simulink model "threephase3level_SVPWM_Bidirectional_C"  (R2024a)
settings: Solver=ode4  StartTime=0.0  StopTime=0.5  FixedStep=1e-6  MaxStep=0.00001  MinStep=0.000001  RelTol=1e-3  EnableMultiTasking=on
libraries: spsIGBTDiodeLib x12, spsDiodeLib x6, spsVoltageMeasurementLib x6, slpidlib x4, spsACVoltageSourceLib x3, spsSeriesRLCBranchLib x3, spsabctoAlphaBetaZeroLib x2, spsAlphaBetaZerotodq0Lib x1, spsControlledVoltageSourceLib x1, spsCurrentMeasurementLib x1, spsGroundLib x1, simulink x1
settings Model: Creator=hp  LastModifiedBy=rkavi
settings SolverCC: ZeroCrossControl=DisableAll  AlgebraicLoopSolver=TrustRegion
settings DataIOCC: LimitDataPoints=on  SaveFormat=Array  ReturnWorkspaceOutputs=off
settings OptimizationCC: LifeSpan=inf
settings DebuggingCC: UnconnectedInputMsg=warning  UnconnectedOutputMsg=warning  UnconnectedLineMsg=warning  SFUnexpectedBacktrackingDiag=warning  SFNoUnconditionalDefaultTransitionDiag=warning  ArithmeticOperatorsInVariantConditions=warning
settings HardwareCC: ProdBitPerPointer=32  ProdBitPerSizeT=32  ProdBitPerPtrDiffT=32  ProdLargestAtomicFloat=None  ProdIntDivRoundTo=Undefined  ProdEndianess=Unspecified  ProdWordSize=32  ProdHWDeviceType=32-bit Generic
settings ModelReferenceCC: EnableRefExpFcnMdlSchedulingChecks=on  PropagateSignalLabelsOutOfModel=off
settings SFSimCC: SimUseLocalCustomCode=off  CustomCodeUndefinedFunction=UseInterfaceOnly
settings RTWCC: RTWUseLocalCustomCode=off  GPUComputeCapability=3.5
settings CodeAppCC: StateflowObjectComments=on
settings GRTTargetCC: TargetLangStandard=C89/C90 (ANSI)
settings ConfigComp: CovMetricSettings=dw  CovSaveCumulativeToWorkspaceVar=on  CovSaveSingleToWorkspaceVar=on  CovExternalEMLEnable=off
settings SimscapeCC: SimscapeNormalizeSystem=off

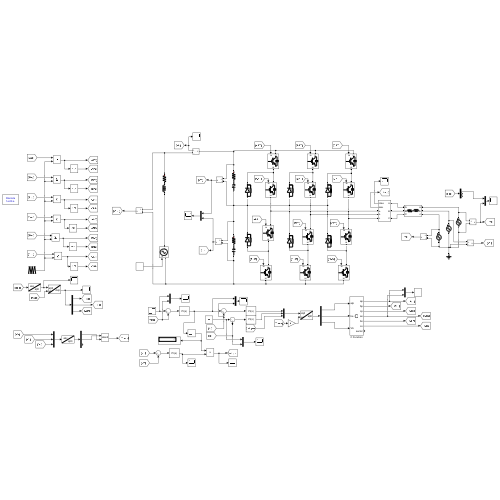
[thumbnail: Simulink's stored preview of the top-level diagram]
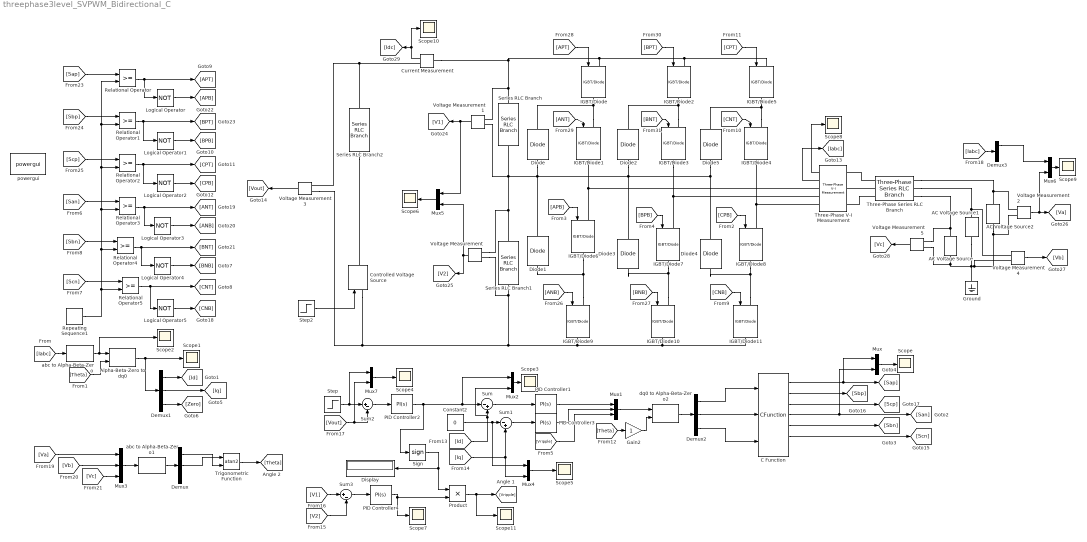
== system threephase3level_SVPWM_Bidirectional_C ==
  AC Voltage Source : spsACVoltageSourceLib/AC Voltage Source  Amplitude=325  Phase=240  Frequency=50  SampleTime=0  Measurements=None  BusType=swing  Pref=10e3  Qref=0  Qmin=-inf  Qmax=+inf
  AC Voltage Source1 : spsACVoltageSourceLib/AC Voltage Source  Amplitude=325  Phase=120  Frequency=50  SampleTime=0  Measurements=None  BusType=swing  Pref=10e3  Qref=0  Qmin=-inf  Qmax=+inf
  AC Voltage Source2 : spsACVoltageSourceLib/AC Voltage Source  Amplitude=325  Phase=0  Frequency=50  SampleTime=0  Measurements=None  BusType=swing  Pref=10e3  Qref=0  Qmin=-inf  Qmax=+inf
  Alpha-Beta-Zero to dq0 : spsAlphaBetaZerotodq0Lib/Alpha-Beta-Zero to dq0  Alignment=Aligned with phase A axis
  C Function : CFunction  OutputCode=|  CodegenOutputCode=|
      OutputCode=|
      | float sec_a=0,sec_b=0,sec_c=0;
      | 	float t_o = 0,ta = 0,tb = 0,tc = 0,tsec = 0;
      | 
      |     sec_a = be;										//Beta;
      | 	sec_b = ((-be/2)+(alp*0.866));			//(-0.5*Beta+(0.866*alpha));
      | 	sec_c = ((-be/2)-(alp*0.866));			//(-0.5*Beta-(0.866*alpha));
      |     
      |     if(sec_a>=0)
      |      {
      |          if(sec_b>=0)
      |        	  {											//	sector 1
      |     		t_o = ((1 - (sec_a+sec_b))/2)-Vb;							//	t_1 = sec_b, t_2 =sec_a
      |     		ta = sec_a+sec_b+(t_o);
      |     		tb  = sec_a+(t_o);
      |     		tc  = (t_o);
      |             tsec = 1;
      |          }
      |        else
      |          {
      |             if(sec_c>=0)												//	sector 3
      |         	{
      |             	t_o = ((1 - (sec_a+sec_c))/2)-Vb;						//	t_1 = sec_a, t_2 =sec_c
      |         		ta = (t_o);
      |         		tb = sec_a+sec_c+(t_o);
      |         		tc = sec_c+(t_o);
      |                 tsec = 3;
      |              }
      |             else
      |             {                                                        //	sector 2
      |         		t_o = ((1 + (sec_c+sec_b))/2)-Vb;					//	t_1 = -sec_c, t_2 =-sec_b
      |         		ta = -sec_c+(t_o);
      |         		tb = -(sec_c+sec_b)+(t_o);
      |         		tc = (t_o);
      |                 tsec = 2;
      |             }
      |        }
      |      }
      |     else
      |        {
      |          if(sec_b>=0)
      |            {
      |                if(sec_c>=0)                                                  //	sector 5
      |         		{
      |                     t_o = ((1 - (sec_c+sec_b))/2)-Vb; 				//	t_1 = sec_c, t_2 =sec_b
      |         		    ta = sec_b+(t_o);
      |         		    tb = (t_o);
      |         		    tc = sec_c+sec_b+(t_o);
      |                     tsec = 5;    
      |                 }
      |            else                                                  //	sector 6
      |         		{
      |                     t_o = ((1 + (sec_a+sec_c))/2)-Vb; 				//	t_1 = -sec_a, t_2 =-sec_c
      |         		    ta = -(sec_a+sec_c)+(t_o);
      |         		    tb = (t_o);
      |         		    tc = -sec_a+(t_o);
      |                     tsec = 6;
      |                 }
      |         }
      |        else
      |            {
      |                if(sec_c>=0)                                      //	sector 4
      |         		{
      |                     t_o = ((1 + (sec_a+sec_b))/2)-Vb;			//	t_1 = -sec_b, t_2 =-sec_a
      |         		    ta = (t_o);
      |         		    tb = -sec_b+(t_o);
      |         		    tc = -(sec_a+sec_b)+(t_o);
      |                     tsec = 4;
      |                }
      |        }
      |     }
      | 
      | if(ta>1)
      | {
      |     ta = 1;
      | }
      | if(tb>1)
      | {
      |     tb = 1;
      | }
      | if(tc>1)
      | {
      |     tc = 1; 
      | }
      | if(ta<0)            
      | {
      |     ta = 0;
      | }
      | if(tb<0)
      | {
      |     tb = 0;
      | }
      | if(tc<0)
      | {
      |     tc = 0;
      | }
      | if(ta>0.5)
      | {
      |         ap = (2*ta)-1;
      |         an = 1;
      | }
      | else
      | {   ap = 0;
      |     an = 2*ta;
      | }
      | 
      | if(tb>0.5)
      | {    bp = (2*tb)-1;
      |     bn = 1;
      | }
      | else
      | {    bp = 0;
      |     bn = 2*tb;
      | }
      | 
      | if(tc>0.5)
      | {    cp = (2*tc)-1;
      |     cn = 1;
      | }
      | else
      | {    cp = 0;
      |     cn = 2*tc;
      | }
      | 
      | sector = tsec;
      CodegenOutputCode=|
      | float sec_a=0,sec_b=0,sec_c=0;
      | 	float t_o = 0,ta = 0,tb = 0,tc = 0,tsec = 0;
      | 
      |     sec_a = be;										//Beta;
      | 	sec_b = ((-be/2)+(alp*0.866));			//(-0.5*Beta+(0.866*alpha));
      | 	sec_c = ((-be/2)-(alp*0.866));			//(-0.5*Beta-(0.866*alpha));
      |     
      |     if(sec_a>=0)
      |      {
      |          if(sec_b>=0)
      |        	  {											//	sector 1
      |     		t_o = ((1 - (sec_a+sec_b))/2)-Vb;							//	t_1 = sec_b, t_2 =sec_a
      |     		ta = sec_a+sec_b+(t_o);
      |     		tb  = sec_a+(t_o);
      |     		tc  = (t_o);
      |             tsec = 1;
      |          }
      |        else
      |          {
      |             if(sec_c>=0)												//	sector 3
      |         	{
      |             	t_o = ((1 - (sec_a+sec_c))/2)-Vb;						//	t_1 = sec_a, t_2 =sec_c
      |         		ta = (t_o);
      |         		tb = sec_a+sec_c+(t_o);
      |         		tc = sec_c+(t_o);
      |                 tsec = 3;
      |              }
      |             else
      |             {                                                        //	sector 2
      |         		t_o = ((1 + (sec_c+sec_b))/2)-Vb;					//	t_1 = -sec_c, t_2 =-sec_b
      |         		ta = -sec_c+(t_o);
      |         		tb = -(sec_c+sec_b)+(t_o);
      |         		tc = (t_o);
      |                 tsec = 2;
      |             }
      |        }
      |      }
      |     else
      |        {
      |          if(sec_b>=0)
      |            {
      |                if(sec_c>=0)                                                  //	sector 5
      |         		{
      |                     t_o = ((1 - (sec_c+sec_b))/2)-Vb; 				//	t_1 = sec_c, t_2 =sec_b
      |         		    ta = sec_b+(t_o);
      |         		    tb = (t_o);
      |         		    tc = sec_c+sec_b+(t_o);
      |                     tsec = 5;    
      |                 }
      |            else                                                  //	sector 6
      |         		{
      |                     t_o = ((1 + (sec_a+sec_c))/2)-Vb; 				//	t_1 = -sec_a, t_2 =-sec_c
      |         		    ta = -(sec_a+sec_c)+(t_o);
      |         		    tb = (t_o);
      |         		    tc = -sec_a+(t_o);
      |                     tsec = 6;
      |                 }
      |         }
      |        else
      |            {
      |                if(sec_c>=0)                                      //	sector 4
      |         		{
      |                     t_o = ((1 + (sec_a+sec_b))/2)-Vb;			//	t_1 = -sec_b, t_2 =-sec_a
      |         		    ta = (t_o);
      |         		    tb = -sec_b+(t_o);
      |         		    tc = -(sec_a+sec_b)+(t_o);
      |                     tsec = 4;
      |                }
      |        }
      |     }
      | 
      | if(ta>1)
      | {
      |     ta = 1;
      | }
      | if(tb>1)
      | {
      |     tb = 1;
      | }
      | if(tc>1)
      | {
      |     tc = 1; 
      | }
      | if(ta<0)            
      | {
      |     ta = 0;
      | }
      | if(tb<0)
      | {
      |     tb = 0;
      | }
      | if(tc<0)
      | {
      |     tc = 0;
      | }
      | if(ta>0.5)
      | {
      |         ap = (2*ta)-1;
      |         an = 1;
      | }
      | else
      | {   ap = 0;
      |     an = 2*ta;
      | }
      | 
      | if(tb>0.5)
      | {    bp = (2*tb)-1;
      |     bn = 1;
      | }
      | else
      | {    bp = 0;
      |     bn = 2*tb;
      | }
      | 
      | if(tc>0.5)
      | {    cp = (2*tc)-1;
      |     cn = 1;
      | }
      | else
      | {    cp = 0;
      |     cn = 2*tc;
      | }
      | 
      | sector = tsec;
  Constant2 : Constant  Value=0
  Controlled Voltage Source : spsControlledVoltageSourceLib/Controlled Voltage Source  Initialize=on  Source_Type=DC  Amplitude=0  Phase=0  Frequency=0  Measurements=None
  Current Measurement : spsCurrentMeasurementLib/Current Measurement  PhasorSimulation=off  OutputType=Complex  PSBequivalent=0
  Demux{,1..3} (4 alike) : Demux  Outputs=3
  Diode{,1..5} (6 alike) : spsDiodeLib/Diode  Ron=0.001  Lon=0  Vf=0.8  IC=0  UseSnubber=off  Rs=500  Cs=250e-9  Measurements=off
  Display : Display
  Gain2 : Gain  OutDataTypeStr=single
  Ground : spsGroundLib/Ground  LConnTagsString=a
  IGBT/Diode{,1..11} (12 alike) : spsIGBTDiodeLib/IGBT//Diode  Ron=1e-3  Rs=1e5  Cs=inf  Measurements=off
  Logical Operator{,1..5} (6 alike) : Logic  Operator=NOT  Inputs=1  AllPortsSameDT=off  OutDataTypeStr=boolean
  Mux{,2,4..7} (6 alike) : Mux  Inputs=2
  Mux1 : Mux  Inputs=3
  Mux3 : Mux  Inputs=3
  PID Controller1 : slpidlib/PID Controller  Controller=PI  Form=Parallel  TimeDomain=Continuous-time  UseExternalTs=off  SampleTime=-1  IntegratorMethod=Forward Euler  FilterMethod=Forward Euler  ControllerParametersSource=internal  P=0.05  I=5  UseKiTs=off  D=0  UseExternalDerivativeSource=off  N=100  UseFilter=on  TunerSelectOption=Transfer Function Based (PID Tuner App)  InitialConditionSource=internal  InitialConditionForIntegrator=0  InitialConditionForFilter=0  DifferentiatorICPrevScaledInput=0  ExternalReset=none  TrackingMode=off  Kt=1  LimitOutput=off  SatLimitsSource=internal  UpperSaturationLimit=inf  LowerSaturationLimit=-inf  LinearizeAsGain=on  AntiWindupMode=none  Kb=1  LimitIntegrator=off  UpperIntegratorSaturationLimit=inf  LowerIntegratorSaturationLimit=-inf  POutMin=[]  POutMax=[]  IOutMin=[]  IOutMax=[]  DOutMin=[]  DOutMax=[]  NOutMin=[]  NOutMax=[]  SumOutDataTypeStr=single  SumOutMin=[]  SumOutMax=[]  SaturationOutMin=[]  SaturationOutMax=[]  PParamMin=[]  PParamMax=[]  IParamMin=[]  IParamMax=[]  DParamMin=[]  DParamMax=[]  NParamMin=[]  NParamMax=[]  KbParamMin=[]  KbParamMax=[]  KtParamMin=[]  KtParamMax=[]  KbOutMin=[]  KbOutMax=[]  KtOutMin=[]  KtOutMax=[]  IntegratorOutMin=[]  IntegratorOutMax=[]  FilterOutMin=[]  FilterOutMax=[]  SumI1OutMin=[]  SumI1OutMax=[]  SumI2OutMin=[]  SumI2OutMax=[]  SumI3OutMin=[]  SumI3OutMax=[]  SumI4OutMin=[]  SumI4OutMax=[]  SumDOutMin=[]  SumDOutMax=[]  DifferentiatorOutMin=[]  DifferentiatorOutMax=[]  FilterDiffOutCoefMin=[]  FilterDiffOutCoefMax=[]  ReciprocalOutMin=[]  ReciprocalOutMax=[]  SumDenOutMin=[]  SumDenOutMax=[]  SumNumOutMin=[]  SumNumOutMax=[]  DivideOutMin=[]  DivideOutMax=[]  UdiffTsProdOutMin=[]  UdiffTsProdOutMax=[]  NTsProdOutMin=[]  NTsProdOutMax=[]  UintegralTsProdOutMin=[]  UintegralTsProdOutMax=[]  UngainTsProdOutMin=[]  UngainTsProdOutMax=[]  ClampingZeroOutDataTypeStr=Inherit: Inherit via back propagation  ClampingZeroOutMin=[]  ClampingZeroOutMax=[]  FilterDenConstantOutDataTypeStr=Inherit: Inherit via back propagation  FilterDenConstantOutMin=[]  FilterDenConstantOutMax=[]  PCopyOutDataTypeStr=Inherit: Inherit via back propagation  PCopyOutMin=[]  PCopyOutMax=[]  NCopyOutDataTypeStr=Inherit: Inherit via back propagation  NCopyOutMin=[]  NCopyOutMax=[]  IntegratorContinuousStateAttributes=''  IntegratorStateMustResolveToSignalObject=off  IntegratorRTWStateStorageClass=Auto  FilterContinuousStateAttributes=''  FilterStateMustResolveToSignalObject=off  FilterRTWStateStorageClass=Auto  ParallelPVariant=InternalParameters  IdealPVariant=Disabled  IVariant=InternalParameters  DVariant=Disabled  IntegratorVariant=Continuous  SatVariant=Disabled  AWVariant=Passthrough  PCopyVariant=Disabled  TRVariant=Disabled  FdbkBlocksVariant=Forward  IdealPFdbkVariant=Disabled  SatFdbkVariant=Disabled  DerivativeFilterVariant=Disabled  NVariant=Disabled  NCopyVariant=Disabled_SignalSpec  FilterICVariant=Disabled  IntegratorICVariant=InternalICs  ExternalResetVariant=Disabled  TRSumVariant=Passthrough  SumFdbkVariant=Disabled  SumVariant=Sum_PI  TsampFilterVariant=InternalTs  TsampNgainVariant=Passthrough  TsampIntegralVariant=Disabled_SignalSpec  ExternalSaturationOutDataTypeStr=Inherit: Same as second input  DerivativeSourceVariant=Disabled
  PID Controller2 : slpidlib/PID Controller  Controller=PI  Form=Parallel  TimeDomain=Continuous-time  UseExternalTs=off  SampleTime=-1  IntegratorMethod=Forward Euler  FilterMethod=Forward Euler  ControllerParametersSource=internal  P=1.0  I=300  UseKiTs=off  D=0  UseExternalDerivativeSource=off  N=100  UseFilter=on  TunerSelectOption=Transfer Function Based (PID Tuner App)  InitialConditionSource=internal  InitialConditionForIntegrator=0  InitialConditionForFilter=0  DifferentiatorICPrevScaledInput=0  ExternalReset=none  TrackingMode=off  Kt=1  LimitOutput=off  SatLimitsSource=internal  UpperSaturationLimit=inf  LowerSaturationLimit=-inf  LinearizeAsGain=on  AntiWindupMode=none  Kb=1  LimitIntegrator=off  UpperIntegratorSaturationLimit=inf  LowerIntegratorSaturationLimit=-inf  POutMin=[]  POutMax=[]  IOutMin=[]  IOutMax=[]  DOutMin=[]  DOutMax=[]  NOutMin=[]  NOutMax=[]  SumOutMin=[]  SumOutMax=[]  SaturationOutMin=[]  SaturationOutMax=[]  PParamMin=[]  PParamMax=[]  IParamMin=[]  IParamMax=[]  DParamMin=[]  DParamMax=[]  NParamMin=[]  NParamMax=[]  KbParamMin=[]  KbParamMax=[]  KtParamMin=[]  KtParamMax=[]  KbOutMin=[]  KbOutMax=[]  KtOutMin=[]  KtOutMax=[]  IntegratorOutMin=[]  IntegratorOutMax=[]  FilterOutMin=[]  FilterOutMax=[]  SumI1OutMin=[]  SumI1OutMax=[]  SumI2OutMin=[]  SumI2OutMax=[]  SumI3OutMin=[]  SumI3OutMax=[]  SumI4OutMin=[]  SumI4OutMax=[]  SumDOutMin=[]  SumDOutMax=[]  DifferentiatorOutMin=[]  DifferentiatorOutMax=[]  FilterDiffOutCoefMin=[]  FilterDiffOutCoefMax=[]  ReciprocalOutMin=[]  ReciprocalOutMax=[]  SumDenOutMin=[]  SumDenOutMax=[]  SumNumOutMin=[]  SumNumOutMax=[]  DivideOutMin=[]  DivideOutMax=[]  UdiffTsProdOutMin=[]  UdiffTsProdOutMax=[]  NTsProdOutMin=[]  NTsProdOutMax=[]  UintegralTsProdOutMin=[]  UintegralTsProdOutMax=[]  UngainTsProdOutMin=[]  UngainTsProdOutMax=[]  ClampingZeroOutDataTypeStr=Inherit: Inherit via back propagation  ClampingZeroOutMin=[]  ClampingZeroOutMax=[]  FilterDenConstantOutDataTypeStr=Inherit: Inherit via back propagation  FilterDenConstantOutMin=[]  FilterDenConstantOutMax=[]  PCopyOutDataTypeStr=Inherit: Inherit via back propagation  PCopyOutMin=[]  PCopyOutMax=[]  NCopyOutDataTypeStr=Inherit: Inherit via back propagation  NCopyOutMin=[]  NCopyOutMax=[]  IntegratorContinuousStateAttributes=''  IntegratorStateMustResolveToSignalObject=off  IntegratorRTWStateStorageClass=Auto  FilterContinuousStateAttributes=''  FilterStateMustResolveToSignalObject=off  FilterRTWStateStorageClass=Auto  ParallelPVariant=InternalParameters  IdealPVariant=Disabled  IVariant=InternalParameters  DVariant=Disabled  IntegratorVariant=Continuous  SatVariant=Disabled  AWVariant=Passthrough  PCopyVariant=Disabled  TRVariant=Disabled  FdbkBlocksVariant=Forward  IdealPFdbkVariant=Disabled  SatFdbkVariant=Disabled  DerivativeFilterVariant=Disabled  NVariant=Disabled  NCopyVariant=Disabled_SignalSpec  FilterICVariant=Disabled  IntegratorICVariant=InternalICs  ExternalResetVariant=Disabled  TRSumVariant=Passthrough  SumFdbkVariant=Disabled  SumVariant=Sum_PI  TsampFilterVariant=InternalTs  TsampNgainVariant=Passthrough  TsampIntegralVariant=Disabled_SignalSpec  ExternalSaturationOutDataTypeStr=Inherit: Same as second input  DerivativeSourceVariant=Disabled
  PID Controller3 : slpidlib/PID Controller  Controller=PI  Form=Parallel  TimeDomain=Continuous-time  UseExternalTs=off  SampleTime=-1  IntegratorMethod=Forward Euler  FilterMethod=Forward Euler  ControllerParametersSource=internal  P=0.05  I=5  UseKiTs=off  D=0  UseExternalDerivativeSource=off  N=100  UseFilter=on  TunerSelectOption=Transfer Function Based (PID Tuner App)  InitialConditionSource=internal  InitialConditionForIntegrator=0  InitialConditionForFilter=0  DifferentiatorICPrevScaledInput=0  ExternalReset=none  TrackingMode=off  Kt=1  LimitOutput=off  SatLimitsSource=internal  UpperSaturationLimit=inf  LowerSaturationLimit=-inf  LinearizeAsGain=on  AntiWindupMode=none  Kb=1  LimitIntegrator=off  UpperIntegratorSaturationLimit=inf  LowerIntegratorSaturationLimit=-inf  POutMin=[]  POutMax=[]  IOutMin=[]  IOutMax=[]  DOutMin=[]  DOutMax=[]  NOutMin=[]  NOutMax=[]  SumOutDataTypeStr=single  SumOutMin=[]  SumOutMax=[]  SaturationOutMin=[]  SaturationOutMax=[]  PParamMin=[]  PParamMax=[]  IParamMin=[]  IParamMax=[]  DParamMin=[]  DParamMax=[]  NParamMin=[]  NParamMax=[]  KbParamMin=[]  KbParamMax=[]  KtParamMin=[]  KtParamMax=[]  KbOutMin=[]  KbOutMax=[]  KtOutMin=[]  KtOutMax=[]  IntegratorOutMin=[]  IntegratorOutMax=[]  FilterOutMin=[]  FilterOutMax=[]  SumI1OutMin=[]  SumI1OutMax=[]  SumI2OutMin=[]  SumI2OutMax=[]  SumI3OutMin=[]  SumI3OutMax=[]  SumI4OutMin=[]  SumI4OutMax=[]  SumDOutMin=[]  SumDOutMax=[]  DifferentiatorOutMin=[]  DifferentiatorOutMax=[]  FilterDiffOutCoefMin=[]  FilterDiffOutCoefMax=[]  ReciprocalOutMin=[]  ReciprocalOutMax=[]  SumDenOutMin=[]  SumDenOutMax=[]  SumNumOutMin=[]  SumNumOutMax=[]  DivideOutMin=[]  DivideOutMax=[]  UdiffTsProdOutMin=[]  UdiffTsProdOutMax=[]  NTsProdOutMin=[]  NTsProdOutMax=[]  UintegralTsProdOutMin=[]  UintegralTsProdOutMax=[]  UngainTsProdOutMin=[]  UngainTsProdOutMax=[]  ClampingZeroOutDataTypeStr=Inherit: Inherit via back propagation  ClampingZeroOutMin=[]  ClampingZeroOutMax=[]  FilterDenConstantOutDataTypeStr=Inherit: Inherit via back propagation  FilterDenConstantOutMin=[]  FilterDenConstantOutMax=[]  PCopyOutDataTypeStr=Inherit: Inherit via back propagation  PCopyOutMin=[]  PCopyOutMax=[]  NCopyOutDataTypeStr=Inherit: Inherit via back propagation  NCopyOutMin=[]  NCopyOutMax=[]  IntegratorContinuousStateAttributes=''  IntegratorStateMustResolveToSignalObject=off  IntegratorRTWStateStorageClass=Auto  FilterContinuousStateAttributes=''  FilterStateMustResolveToSignalObject=off  FilterRTWStateStorageClass=Auto  ParallelPVariant=InternalParameters  IdealPVariant=Disabled  IVariant=InternalParameters  DVariant=Disabled  IntegratorVariant=Continuous  SatVariant=Disabled  AWVariant=Passthrough  PCopyVariant=Disabled  TRVariant=Disabled  FdbkBlocksVariant=Forward  IdealPFdbkVariant=Disabled  SatFdbkVariant=Disabled  DerivativeFilterVariant=Disabled  NVariant=Disabled  NCopyVariant=Disabled_SignalSpec  FilterICVariant=Disabled  IntegratorICVariant=InternalICs  ExternalResetVariant=Disabled  TRSumVariant=Passthrough  SumFdbkVariant=Disabled  SumVariant=Sum_PI  TsampFilterVariant=InternalTs  TsampNgainVariant=Passthrough  TsampIntegralVariant=Disabled_SignalSpec  ExternalSaturationOutDataTypeStr=Inherit: Same as second input  DerivativeSourceVariant=Disabled
  PID Controller4 : slpidlib/PID Controller  Controller=PI  Form=Parallel  TimeDomain=Continuous-time  UseExternalTs=off  SampleTime=-1  IntegratorMethod=Forward Euler  FilterMethod=Forward Euler  ControllerParametersSource=internal  P=0.001  I=0.07  UseKiTs=off  D=0  UseExternalDerivativeSource=off  N=100  UseFilter=on  TunerSelectOption=Transfer Function Based (PID Tuner App)  InitialConditionSource=internal  InitialConditionForIntegrator=0  InitialConditionForFilter=0  DifferentiatorICPrevScaledInput=0  ExternalReset=none  TrackingMode=off  Kt=1  LimitOutput=off  SatLimitsSource=internal  UpperSaturationLimit=inf  LowerSaturationLimit=-inf  LinearizeAsGain=on  AntiWindupMode=none  Kb=1  LimitIntegrator=off  UpperIntegratorSaturationLimit=inf  LowerIntegratorSaturationLimit=-inf  POutMin=[]  POutMax=[]  IOutMin=[]  IOutMax=[]  DOutMin=[]  DOutMax=[]  NOutMin=[]  NOutMax=[]  SumOutMin=[]  SumOutMax=[]  SaturationOutMin=[]  SaturationOutMax=[]  PParamMin=[]  PParamMax=[]  IParamMin=[]  IParamMax=[]  DParamMin=[]  DParamMax=[]  NParamMin=[]  NParamMax=[]  KbParamMin=[]  KbParamMax=[]  KtParamMin=[]  KtParamMax=[]  KbOutMin=[]  KbOutMax=[]  KtOutMin=[]  KtOutMax=[]  IntegratorOutMin=[]  IntegratorOutMax=[]  FilterOutMin=[]  FilterOutMax=[]  SumI1OutMin=[]  SumI1OutMax=[]  SumI2OutMin=[]  SumI2OutMax=[]  SumI3OutMin=[]  SumI3OutMax=[]  SumI4OutMin=[]  SumI4OutMax=[]  SumDOutMin=[]  SumDOutMax=[]  DifferentiatorOutMin=[]  DifferentiatorOutMax=[]  FilterDiffOutCoefMin=[]  FilterDiffOutCoefMax=[]  ReciprocalOutMin=[]  ReciprocalOutMax=[]  SumDenOutMin=[]  SumDenOutMax=[]  SumNumOutMin=[]  SumNumOutMax=[]  DivideOutMin=[]  DivideOutMax=[]  UdiffTsProdOutMin=[]  UdiffTsProdOutMax=[]  NTsProdOutMin=[]  NTsProdOutMax=[]  UintegralTsProdOutMin=[]  UintegralTsProdOutMax=[]  UngainTsProdOutMin=[]  UngainTsProdOutMax=[]  ClampingZeroOutDataTypeStr=Inherit: Inherit via back propagation  ClampingZeroOutMin=[]  ClampingZeroOutMax=[]  FilterDenConstantOutDataTypeStr=Inherit: Inherit via back propagation  FilterDenConstantOutMin=[]  FilterDenConstantOutMax=[]  PCopyOutDataTypeStr=Inherit: Inherit via back propagation  PCopyOutMin=[]  PCopyOutMax=[]  NCopyOutDataTypeStr=Inherit: Inherit via back propagation  NCopyOutMin=[]  NCopyOutMax=[]  IntegratorContinuousStateAttributes=''  IntegratorStateMustResolveToSignalObject=off  IntegratorRTWStateStorageClass=Auto  FilterContinuousStateAttributes=''  FilterStateMustResolveToSignalObject=off  FilterRTWStateStorageClass=Auto  ParallelPVariant=InternalParameters  IdealPVariant=Disabled  IVariant=InternalParameters  DVariant=Disabled  IntegratorVariant=Continuous  SatVariant=Disabled  AWVariant=Passthrough  PCopyVariant=Disabled  TRVariant=Disabled  FdbkBlocksVariant=Forward  IdealPFdbkVariant=Disabled  SatFdbkVariant=Disabled  DerivativeFilterVariant=Disabled  NVariant=Disabled  NCopyVariant=Disabled_SignalSpec  FilterICVariant=Disabled  IntegratorICVariant=InternalICs  ExternalResetVariant=Disabled  TRSumVariant=Passthrough  SumFdbkVariant=Disabled  SumVariant=Sum_PI  TsampFilterVariant=InternalTs  TsampNgainVariant=Passthrough  TsampIntegralVariant=Disabled_SignalSpec  ExternalSaturationOutDataTypeStr=Inherit: Same as second input  DerivativeSourceVariant=Disabled
  Product : Product  OutDataTypeStr=single
  Relational Operator{,1..5} (6 alike) : RelationalOperator  OutDataTypeStr=boolean  InputSameDT=off
  Repeating Sequence1 : simulink/Sources/Repeating Sequence  rep_seq_t=[0 0.5 1]/5000  rep_seq_y=[0 1 0]
  Scope{,1..11} (12 alike) : Scope
  Series RLC Branch : spsSeriesRLCBranchLib/Series RLC Branch  LConnTagsString=__new0  RConnTagsString=__new0  BranchType=RC  Resistance=1e-6  Inductance=1e-3  SetiL0=off  InitialCurrent=0  Capacitance=3300e-6  Setx0=on  InitialVoltage=325  Measurements=None
  Series RLC Branch1 : spsSeriesRLCBranchLib/Series RLC Branch  LConnTagsString=__new0  RConnTagsString=__new0  BranchType=RC  Resistance=1e-6  Inductance=1e-3  SetiL0=off  InitialCurrent=0  Capacitance=3300e-6  Setx0=on  InitialVoltage=325  Measurements=None
  Series RLC Branch2 : spsSeriesRLCBranchLib/Series RLC Branch  LConnTagsString=__new0  RConnTagsString=__new0  BranchType=RL  Resistance=10  Inductance=1e-3  SetiL0=off  InitialCurrent=0  Capacitance=1e-6  Setx0=off  InitialVoltage=0  Measurements=None
  Sign : Signum
  Step : Step  Time=0.1  Before=800  After=800  SampleTime=0
  Step2 : Step  Time=0.15  Before=-1000  After=1000  SampleTime=0
  Sum : Sum  Inputs=|-+
  Sum1 : Sum  Inputs=|-+
  Sum2 : Sum  Inputs=|+-
  Sum3 : Sum  Inputs=|+-
  Three-Phase Series RLC Branch : spsThreePhaseSeriesRLCBranchLib/Three-Phase Series RLC Branch  LConnTagsString=A|B|C  RConnTagsString=A|B|C  BranchType=RL  Resistance=5e-6  Inductance=1e-3  Capacitance=1e-6  Measurements=None
  Three-Phase V-I Measurement : spsThreePhaseVIMeasurementLib/Three-Phase V-I Measurement  VoltageMeasurement=phase-to-phase  SetLabelV=off  LabelV=Vabc  Vpu=off  VpuLL=off  CurrentMeasurement=yes  SetLabelI=off  LabelI=Iabc  Ipu=off  Pbase=100e6  Vbase=500e3  OutputType=Complex  PhasorSimulation=off  PSBequivalent=0
  Trigonometric Function : Trigonometry  Operator=atan2
  Voltage Measurement{,1..5} (6 alike) : spsVoltageMeasurementLib/Voltage Measurement  PhasorSimulation=off  OutputType=Complex  PSBequivalent=0
  abc to Alpha-Beta-Zero : spsabctoAlphaBetaZeroLib/abc to Alpha-Beta-Zero
  abc to Alpha-Beta-Zero1 : spsabctoAlphaBetaZeroLib/abc to Alpha-Beta-Zero
  dq0 to Alpha-Beta-Zero2 : spsdq0toAlphaBetaZeroLib/dq0 to Alpha-Beta-Zero  Alignment=Aligned with phase A axis
  powergui : sps_lib/powergui  Priority=1  SimulationMode=Discrete  SampleTime=1e-6  frequency=60  Iterations=50  frequencyindice=0  Pbase=100e6  ErrMax=1e-4  UnitsV=kV  UnitsW=MW  buscounter=0  FunctionMessages=off  echomessages=off  EnableUseOfTLC=off  CurrentSourceSwitches=off  DisableSnubberDevices=off  DisableRonSwitches=off  DisableVfSwitches=off  DisplayEquations=off  AutomaticDiscreteSolvers=off  SolverType=Tustin/Backward Euler (TBE)  Interpol=off  ExternalGateDelay=off  methode=off  Ts=100  x0status=blocks  SPID=off  SwTol=0  HookPort=off  NonlinearTolerance=1e-4  nMaxIteration=100  ContinueOnMaxIteration=off  RestoreLinks=warning  ResistiveCurrentMeasurement=off  Frange=[0:2:500]  Ylog=off  Xlog=on  ShowGrid=off  save=off  variable=ZData  structure=0  ZoomFFT=off  StartTime=0.0  cycles=1  DisplayStyle=1  fundamental=60  FreqAxis=off  MaxFrequency=1000  frequencyindicesteady=1  RmsSteady=1  display=off
  wires:
  [Iabc] -> abc to Alpha-Beta-Zero/1
  Alpha-Beta-Zero to dq0/1 -> Demux1/1, Scope1/1
  abc to Alpha-Beta-Zero/1 -> Scope2/1, Alpha-Beta-Zero to dq0/1
  [Theta] -> Alpha-Beta-Zero to dq0/2
  Demux1/1 -> [Id]
  Demux1/2 -> [Iq]
  Demux1/3 -> [Zero]
  dq0 to Alpha-Beta-Zero2/1 -> Demux2/1
  Demux2/3 -> C Function/3
  [Theta] -> Gain2/1
  Gain2/1 -> dq0 to Alpha-Beta-Zero2/2
  Mux1/1 -> dq0 to Alpha-Beta-Zero2/1
  Sum/1 -> PID Controller1/1
  Sum1/1 -> PID Controller3/1
  Mux2/1 -> Scope3/1
  [Iq] -> Mux4/2, Sum1/2
  Mux4/1 -> Scope5/1
  [Id] -> Mux2/2, Sum/2
  PID Controller1/1 -> Mux1/1
  PID Controller3/1 -> Mux1/2
  C Function/1 -> Mux/1, [Sap]
  C Function/2 -> [Sbp]
  C Function/3 -> [Scp]
  C Function/4 -> [San], Mux/2
  C Function/5 -> [Sbn]
  C Function/6 -> [Scn]
  Mux/1 -> Scope/1
  Demux2/1 -> C Function/1
  Demux2/2 -> C Function/2
  [Sap] -> Relational Operator/1
  [Sbp] -> Relational Operator1/1
  [Scp] -> Relational Operator2/1
  Relational Operator/1 -> Logical Operator/1, [APT]
  Logical Operator/1 -> [APB]
  Relational Operator1/1 -> Logical Operator1/1, [BPT]
  Logical Operator1/1 -> [BPB]
  Relational Operator2/1 -> Logical Operator2/1, [CPT]
  Logical Operator2/1 -> [CPB]
  [San] -> Relational Operator3/1
  Repeating Sequence1/1 -> Relational Operator5/2, Relational Operator4/2, Relational Operator3/2, Relational Operator2/2, Relational Operator/2, Relational Operator1/2
  [Sbn] -> Relational Operator4/1
  [Scn] -> Relational Operator5/1
  Relational Operator3/1 -> Logical Operator3/1, [ANT]
  Logical Operator3/1 -> [ANB]
  Relational Operator4/1 -> Logical Operator4/1, [BNT]
  Logical Operator4/1 -> [BNB]
  Relational Operator5/1 -> [CNT], Logical Operator5/1
  Logical Operator5/1 -> [CNB]
  [CPT] -> IGBT/Diode5/1
  [CNT] -> IGBT/Diode4/1
  [BPT] -> IGBT/Diode2/1
  [BNT] -> IGBT/Diode3/1
  [APT] -> IGBT/Diode/1
  [ANT] -> IGBT/Diode1/1
  [CPB] -> IGBT/Diode8/1
  [BPB] -> IGBT/Diode7/1
  [APB] -> IGBT/Diode6/1
  Voltage Measurement/1 -> Mux5/2, [V2]
  [BNB] -> IGBT/Diode10/1
  [ANB] -> IGBT/Diode9/1
  [CNB] -> IGBT/Diode11/1
  Three-Phase V-I Measurement/2 -> [Iabc]
  Trigonometric Function/1 -> [Theta]
  Mux3/1 -> abc to Alpha-Beta-Zero1/1
  abc to Alpha-Beta-Zero1/1 -> Demux/1
  Demux/2 -> Trigonometric Function/1
  Demux/1 -> Trigonometric Function/2
  Sum2/1 -> PID Controller2/1
  Step/1 -> Mux7/1, Sum2/1
  [Vout] -> Mux7/2, Sum2/2
  Voltage Measurement3/1 -> [Vout]
  Voltage Measurement1/1 -> Mux5/1, [V1]
  [V1] -> Sum3/1
  [V2] -> Sum3/2
  Constant2/1 -> Mux4/1, Sum1/1
  Mux5/1 -> Scope6/1
  Three-Phase V-I Measurement/1 -> Scope8/1
  PID Controller4/1 -> Product/2, Scope7/1
  Sum3/1 -> PID Controller4/1
  [Vripple] -> Mux1/3
  Mux6/1 -> Scope9/1
  [Iabc] -> Demux3/1
  Demux3/1 -> Mux6/1
  Voltage Measurement2/1 -> [Va], Mux6/2
  Voltage Measurement4/1 -> [Vb]
  Voltage Measurement5/1 -> [Vc]
  [Va] -> Mux3/1
  [Vb] -> Mux3/2
  [Vc] -> Mux3/3
  Current Measurement/1 -> Scope10/1, [Idc]
  PID Controller2/1 -> Sign/1, Mux2/1, Sum/1
  Step2/1 -> Controlled Voltage Source/1
  Product/1 -> Scope11/1, [Vripple]
  Sign/1 -> Display/1, Product/1
  Mux7/1 -> Scope4/1
  connections:
  IGBT/Diode3/RConn1 -- IGBT/Diode7/LConn1 -- Three-Phase V-I Measurement/RConn2
  IGBT/Diode10/RConn1 -- IGBT/Diode11/RConn1 -- Controlled Voltage Source/LConn1 -- Voltage Measurement3/LConn2 -- Voltage Measurement/LConn2 -- Series RLC Branch1/RConn1 -- IGBT/Diode9/RConn1
  IGBT/Diode4/LConn1 -- IGBT/Diode5/RConn1 -- Diode5/RConn1
  IGBT/Diode3/LConn1 -- IGBT/Diode2/RConn1 -- Diode2/RConn1
  IGBT/Diode5/LConn1 -- IGBT/Diode2/LConn1 -- Current Measurement/LConn1 -- Series RLC Branch/LConn1 -- Voltage Measurement1/LConn1 -- IGBT/Diode/LConn1
  IGBT/Diode1/LConn1 -- IGBT/Diode/RConn1 -- Diode/RConn1
  IGBT/Diode8/LConn1 -- Three-Phase V-I Measurement/RConn3 -- IGBT/Diode4/RConn1
  Series RLC Branch/RConn1 -- Series RLC Branch1/LConn1 -- Voltage Measurement/LConn1 -- Diode5/LConn1 -- Diode4/RConn1 -- Diode2/LConn1 -- Diode3/RConn1 -- Diode/LConn1 -- Diode1/RConn1 -- Voltage Measurement1/LConn2
  IGBT/Diode6/LConn1 -- Three-Phase V-I Measurement/RConn1 -- IGBT/Diode1/RConn1
  IGBT/Diode10/LConn1 -- IGBT/Diode7/RConn1 -- Diode3/LConn1
  IGBT/Diode11/LConn1 -- IGBT/Diode8/RConn1 -- Diode4/LConn1
  IGBT/Diode9/LConn1 -- IGBT/Diode6/RConn1 -- Diode1/LConn1
  Three-Phase Series RLC Branch/LConn2 -- Three-Phase V-I Measurement/LConn2
  Three-Phase Series RLC Branch/LConn3 -- Three-Phase V-I Measurement/LConn3
  Three-Phase Series RLC Branch/LConn1 -- Three-Phase V-I Measurement/LConn1
  AC Voltage Source2/LConn1 -- Voltage Measurement2/LConn2 -- Voltage Measurement4/LConn2 -- Ground/LConn1 -- AC Voltage Source1/LConn1 -- Voltage Measurement5/LConn2 -- AC Voltage Source/LConn1
  Three-Phase Series RLC Branch/RConn3 -- Voltage Measurement5/LConn1 -- AC Voltage Source/RConn1
  Three-Phase Series RLC Branch/RConn2 -- Voltage Measurement4/LConn1 -- AC Voltage Source1/RConn1
  Three-Phase Series RLC Branch/RConn1 -- Voltage Measurement2/LConn1 -- AC Voltage Source2/RConn1
  Current Measurement/RConn1 -- Series RLC Branch2/LConn1 -- Voltage Measurement3/LConn1
  Series RLC Branch2/RConn1 -- Controlled Voltage Source/RConn1
